simulink model "MoWiTO_OL"  (Simulink 8.6)
settings: Solver=ode4  StartTime=0.0  StopTime=TMax  FixedStep=DT  MaxStep=DT  RelTol=1e-3
undefined symbols (not defined in the file or in its folder): DT, OutList, strmatch, TurbParams
settings Model: Creator=bjonkman  LastModifiedBy=misi9170
settings DataIOCC: SaveOutput=off  SaveTime=off  SignalLoggingName=sigsOut
settings DebuggingCC: SaveWithParameterizedLinksMsg=none  SignalResolutionControl=TryResolveAllWithWarning  SolverPrmCheckMsg=none  MultiTaskDSMMsg=warning  MultiTaskCondExecSysMsg=none  FcnCallInpInsideContextMsg=EnableAllAsWarning
settings HardwareCC: TargetUnknown=on

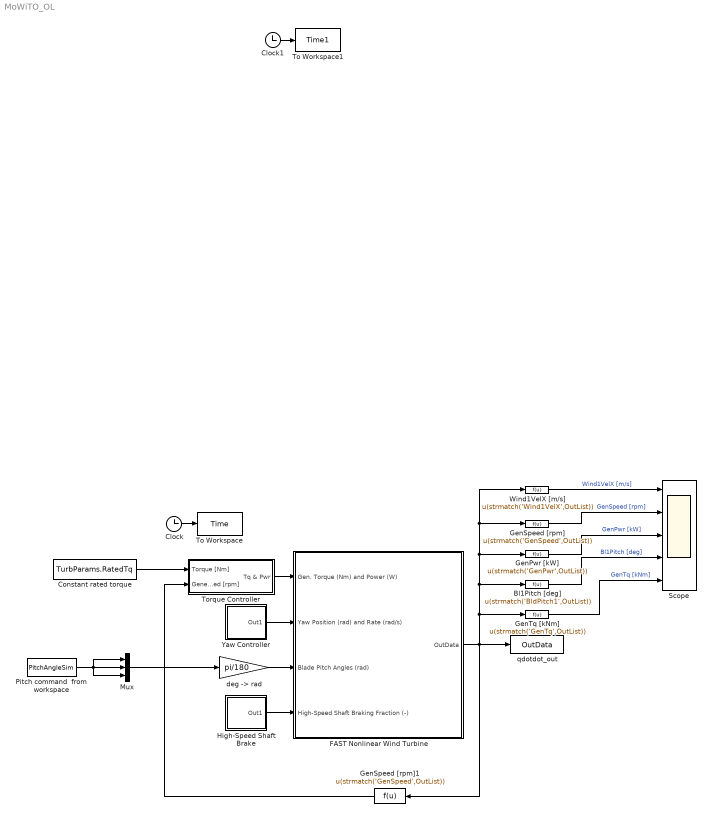
== system MoWiTO_OL ==
  Bl1Pitch [deg] : Fcn  Expr=u(strmatch('BldPitch1',OutList))
  Clock : Clock
  Clock1 : Clock
  Constant rated torque : Constant  Value=TurbParams.RatedTq
  FAST Nonlinear Wind Turbine : Subsystem  mask(FAST Nonlinear Wind Turbine){}
      mask help: This block contains the FAST S-Function.
      mask init:
      | clear FAST_SFunc
  GenPwr [kW] : Fcn  Expr=u(strmatch('GenPwr',OutList))
  GenSpeed [rpm] : Fcn  Expr=u(strmatch('GenSpeed',OutList))
  GenSpeed [rpm]1 : Fcn  Expr=u(strmatch('GenSpeed',OutList))
  GenTq [kNm] : Fcn  Expr=u(strmatch('GenTq',OutList))
  High-Speed Shaft Brake : Subsystem
  Mux : Mux  Inputs=3
  Pitch command  from workspace : FromWorkspace  VariableName=PitchAngleSim  SampleTime=DT
  Scope : Scope  NumInputPorts=5
  To Workspace : ToWorkspace  VariableName=Time  SampleTime=-1
  To Workspace1 : ToWorkspace  VariableName=Time1  SampleTime=-1
  Torque Controller : Subsystem
  Wind1VelX [m/s] : Fcn  Expr=u(strmatch('Wind1VelX',OutList))
  Yaw Controller : Subsystem
  "deg -> rad" : Gain  Gain=pi/180
  qdotdot_out : ToWorkspace  VariableName=OutData  SampleTime=-1
  wires:
  Clock/1 -> To Workspace/1
  FAST Nonlinear Wind Turbine/1(OutData) -> GenSpeed [rpm]1/1, GenTq [kNm]/1, Bl1Pitch [deg]/1, GenPwr [kW]/1, GenSpeed [rpm]/1, Wind1VelX [m/s]/1, qdotdot_out/1
  Torque Controller/1(Tq & Pwr) -> FAST Nonlinear Wind Turbine/1(Gen. Torque (Nm) and Power (W))
  Yaw Controller/1(Out1) -> FAST Nonlinear Wind Turbine/2(Yaw Position (rad) and Rate (rad/s))
  High-Speed Shaft Brake/1(Out1) -> FAST Nonlinear Wind Turbine/4(High-Speed Shaft Braking Fraction (-))
  Constant rated torque/1 -> Torque Controller/1(Torque [Nm])
  Wind1VelX [m/s]/1 -> Scope/1  "Wind1VelX [m/s]"
  GenSpeed [rpm]/1 -> Scope/2  "GenSpeed [rpm]"
  GenPwr [kW]/1 -> Scope/3  "GenPwr [kW]"
  Bl1Pitch [deg]/1 -> Scope/4  "Bl1Pitch [deg]"
  GenTq [kNm]/1 -> Scope/5  "GenTq [kNm]"
  GenSpeed [rpm]1/1 -> Torque Controller/2(Generator speed [rpm])
  Clock1/1 -> To Workspace1/1
  Pitch command  from workspace/1 -> Mux/3, Mux/1, Mux/2
  Mux/1 -> "deg -> rad"/1
  "deg -> rad"/1 -> FAST Nonlinear Wind Turbine/3(Blade Pitch Angles (rad))

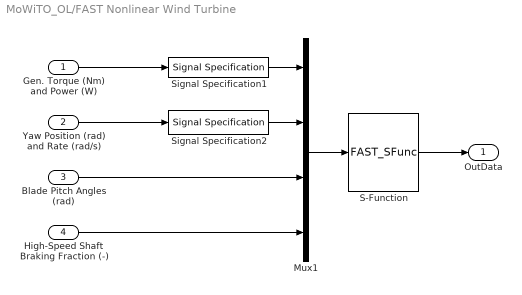
== system MoWiTO_OL/FAST Nonlinear Wind Turbine ==
  Gen. Torque (Nm) and Power (W) : Inport
  Yaw Position (rad) and Rate (rad/s) : Inport  Port=2
  Blade Pitch Angles (rad) : Inport  Port=3
  High-Speed Shaft Braking Fraction (-) : Inport  Port=4
  Mux1 : Mux
  S-Function : S-Function  FunctionName=FAST_SFunc  Parameters=FAST_InputFileName, TMax, 0  SFunctionDeploymentMode=off  EnableBusSupport=off
  Signal Specification1 : SignalSpecification  OutDataTypeStr=double  Dimensions=2
  Signal Specification2 : SignalSpecification  OutDataTypeStr=double  Dimensions=2
  OutData : Outport
  wires:
  Gen. Torque (Nm) and Power (W)/1 -> Signal Specification1/1
  S-Function/1 -> OutData/1
  Mux1/1 -> S-Function/1
  Blade Pitch Angles (rad)/1 -> Mux1/3
  Yaw Position (rad) and Rate (rad/s)/1 -> Signal Specification2/1
  Signal Specification1/1 -> Mux1/1
  Signal Specification2/1 -> Mux1/2
  High-Speed Shaft Braking Fraction (-)/1 -> Mux1/4

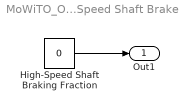
== system MoWiTO_OL/High-Speed Shaft Brake ==
  High-Speed Shaft Braking Fraction : Constant  Value=0
  Out1 : Outport
  wires:
  High-Speed Shaft Braking Fraction/1 -> Out1/1

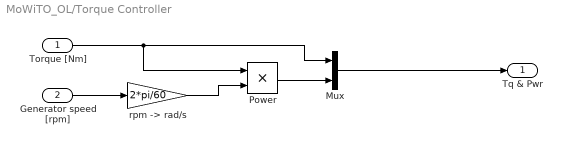
== system MoWiTO_OL/Torque Controller ==
  Torque [Nm] : Inport
  Generator speed [rpm] : Inport  Port=2
  Mux : Mux  Inputs=2
  Power : Product
  "rpm -> rad/s" : Gain  Gain=2*pi/60
  Tq & Pwr : Outport
  wires:
  Mux/1 -> Tq & Pwr/1
  Torque [Nm]/1 -> Power/1, Mux/1
  Power/1 -> Mux/2
  Generator speed [rpm]/1 -> "rpm -> rad/s"/1
  "rpm -> rad/s"/1 -> Power/2

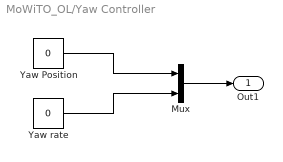
== system MoWiTO_OL/Yaw Controller ==
  Mux : Mux  Inputs=2
  Yaw Position : Constant  Value=0
  Yaw rate : Constant  Value=0
  Out1 : Outport
  wires:
  Mux/1 -> Out1/1
  Yaw Position/1 -> Mux/1
  Yaw rate/1 -> Mux/2
